simulink model "Motor"  (R2021b)
settings: Solver=VariableStepAuto  StartTime=0.0  StopTime=10.0  RelTol=1e-3
model workspace (MAT data in the model file):
  J = 6.5e-07
  Kt = 0.00255
  Kv = 0.00255
  L = 0.000117
  R = 0.117
  b = 2.415e-06
libraries: simulink x2
settings Model: Creator=aakas  LastModifiedBy=aakas

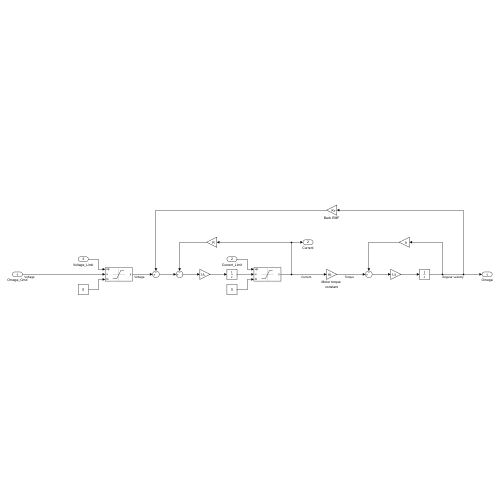
[thumbnail: Simulink's stored preview of the top-level diagram]
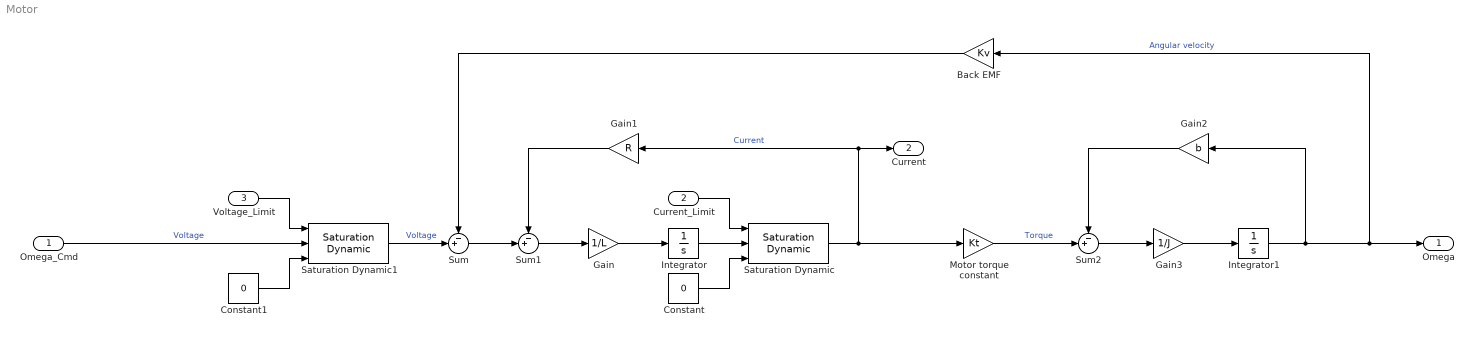
== system Motor ==
  Omega_Cmd : Inport
  Current_Limit : Inport  Port=2
  Voltage_Limit : Inport  Port=3
  Back EMF : Gain  Gain=Kv
  Constant : Constant  Value=0
  Constant1 : Constant  Value=0
  Gain : Gain  Gain=1/L
  Gain1 : Gain  Gain=R
  Gain2 : Gain  Gain=b
  Gain3 : Gain  Gain=1/J
  Integrator : Integrator
  Integrator1 : Integrator
  Motor torque constant : Gain  Gain=Kt
  Saturation Dynamic : simulink/Discontinuities/Saturation Dynamic  OutMin=[]  OutMax=[]  OutDataTypeStr=Inherit: Same as second input  OutDataType=fixdt(1, 16)  OutScaling=2^-10  DoSatur=off
  Saturation Dynamic1 : simulink/Discontinuities/Saturation Dynamic  OutMin=[]  OutMax=[]  OutDataTypeStr=Inherit: Same as second input  OutDataType=fixdt(1, 16)  OutScaling=2^-10  DoSatur=off
  Sum : Sum  Inputs=-+|
  Sum1 : Sum  Inputs=-+|
  Sum2 : Sum  Inputs=-+|
  Omega : Outport
  Current : Outport  Port=2
  wires:
  Saturation Dynamic1/1 -> Sum/2  "Voltage"
  Sum/1 -> Sum1/2
  Sum1/1 -> Gain/1
  Gain/1 -> Integrator/1
  Saturation Dynamic/1 -> Current/1, Gain1/1, Motor torque constant/1  "Current"
  Motor torque constant/1 -> Sum2/2  "Torque"
  Sum2/1 -> Gain3/1
  Gain3/1 -> Integrator1/1
  Integrator1/1 -> Gain2/1, Back EMF/1, Omega/1  "Angular velocity"
  Back EMF/1 -> Sum/1
  Gain2/1 -> Sum2/1
  Gain1/1 -> Sum1/1
  Integrator/1 -> Saturation Dynamic/2
  Current_Limit/1 -> Saturation Dynamic/1
  Constant/1 -> Saturation Dynamic/3
  Constant1/1 -> Saturation Dynamic1/3
  Voltage_Limit/1 -> Saturation Dynamic1/1
  Omega_Cmd/1 -> Saturation Dynamic1/2  "Voltage"
